simulink model "BLDC_Mathematical_Model"  (R2015a)
settings: Solver=ode45  StartTime=0.0  StopTime=1
values from neighbouring files (symbols this model uses):
  B = 2e-3    (= 0.002)    [BLDC_Mathematical_Model_Script.m]
  J = 5.5e-3    (= 0.0055)    [BLDC_Mathematical_Model_Script.m]
  Ke = 1    [BLDC_Mathematical_Model_Script.m]
  Kt = 1    [BLDC_Mathematical_Model_Script.m]
  L = 9.4e-3    (= 0.0094)    [BLDC_Mathematical_Model_Script.m]
  P = 4    [BLDC_Mathematical_Model_Script.m]
  phi_m = 0.2158    [BLDC_Mathematical_Model_Script.m]
  R = 1.43    [BLDC_Mathematical_Model_Script.m]
  trap = 0.2    [BLDC_Mathematical_Model_Script.m]
settings Model: Creator=Koustubh  LastModifiedBy=Koustubh

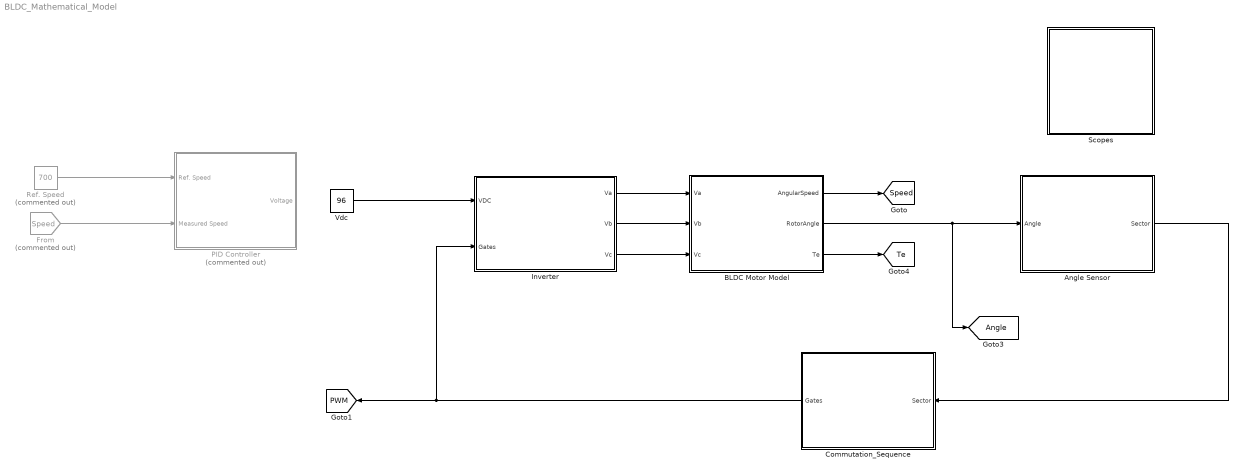
== system BLDC_Mathematical_Model ==
  Angle Sensor : Subsystem
  BLDC Motor Model : Subsystem
      mask Display: image(imread('F:\VAC_2003_MATLAB_Simulink\Practice\BLDC_Mathematical_Model\BLDC_Motor.jpg'))
  Commutation_Sequence : Subsystem
  From : From  Commented=on  GotoTag=Speed  TagVisibility=global
  Inverter : Subsystem
  "PID Controller " : Subsystem  Commented=on
  Ref. Speed : Constant  Commented=on  Value=700
  Scopes : Subsystem
  Vdc : Constant  Value=96
  tag scope: Angle=global, PWM=global, Speed=global, Te=global
  wires:
  BLDC Motor Model/1(AngularSpeed) -> [Speed]
  BLDC Motor Model/2(RotorAngle) -> [Angle], Angle Sensor/1(Angle)
  Angle Sensor/1(Sector) -> Commutation_Sequence/1(Sector)
  Inverter/1(Va) -> BLDC Motor Model/1(Va)
  Inverter/2(Vb) -> BLDC Motor Model/2(Vb)
  Inverter/3(Vc) -> BLDC Motor Model/3(Vc)
  Commutation_Sequence/1(Gates) -> Inverter/2(Gates), [PWM]
  BLDC Motor Model/3(Te) -> [Te]
  From/1 -> "PID Controller "/2(Measured Speed)
  Ref. Speed/1 -> "PID Controller "/1(Ref. Speed)
  Vdc/1 -> Inverter/1(VDC)

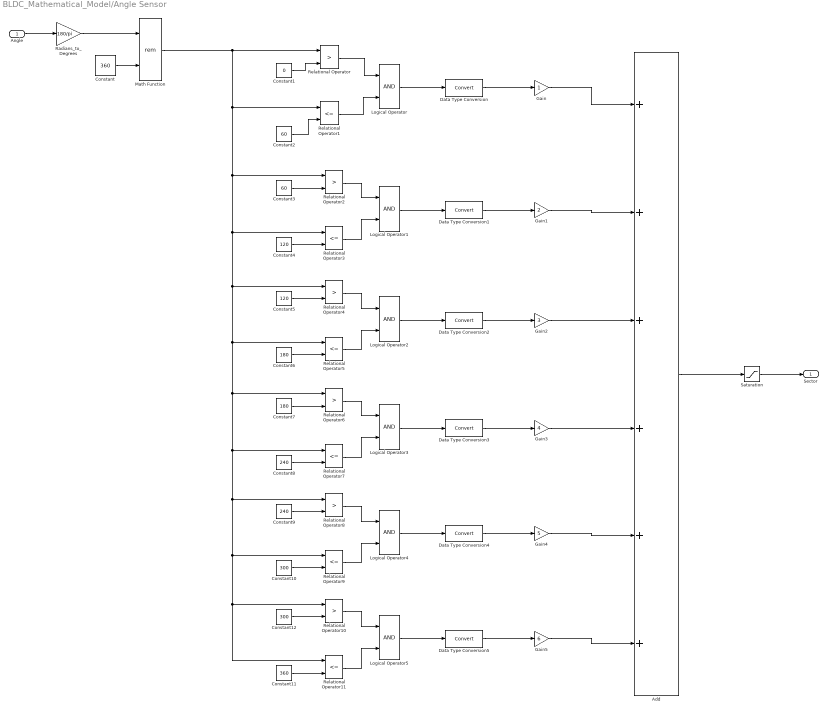
== system BLDC_Mathematical_Model/Angle Sensor ==
  Angle : Inport
  Add : Sum  Inputs=6
  Constant : Constant  Value=360
  Constant1 : Constant  Value=0
  Constant10 : Constant  Value=300
  Constant11 : Constant  Value=360
  Constant12 : Constant  Value=300
  Constant2 : Constant  Value=60
  Constant3 : Constant  Value=60
  Constant4 : Constant  Value=120
  Constant5 : Constant  Value=120
  Constant6 : Constant  Value=180
  Constant7 : Constant  Value=180
  Constant8 : Constant  Value=240
  Constant9 : Constant  Value=240
  Data Type Conversion{,1..5} (6 alike) : DataTypeConversion
  Gain : Gain
  Gain1 : Gain  Gain=2
  Gain2 : Gain  Gain=3
  Gain3 : Gain  Gain=4
  Gain4 : Gain  Gain=5
  Gain5 : Gain  Gain=6
  Logical Operator{,1..5} (6 alike) : Logic  AllPortsSameDT=off  OutDataTypeStr=boolean
  Math Function : Math  Operator=rem  SaturateOnIntegerOverflow=on
  Radians_to_Degrees : Gain  Gain=180/pi
  Relational Operator{,2,4,6,8,10} (6 alike) : RelationalOperator  Operator=>  OutDataTypeStr=boolean
  Relational Operator{1,3,5,7,9,11} (6 alike) : RelationalOperator  Operator=<=  OutDataTypeStr=boolean
  Saturation : Saturate  UpperLimit=6  LowerLimit=1
  Sector : Outport
  wires:
  Constant/1 -> Math Function/2
  Constant1/1 -> Relational Operator/2
  Constant2/1 -> Relational Operator1/2
  Relational Operator/1 -> Logical Operator/1
  Relational Operator1/1 -> Logical Operator/2
  Constant3/1 -> Relational Operator2/2
  Constant4/1 -> Relational Operator3/2
  Relational Operator2/1 -> Logical Operator1/1
  Relational Operator3/1 -> Logical Operator1/2
  Logical Operator/1 -> Data Type Conversion/1
  Data Type Conversion/1 -> Gain/1
  Logical Operator1/1 -> Data Type Conversion1/1
  Data Type Conversion1/1 -> Gain1/1
  Constant5/1 -> Relational Operator4/2
  Constant6/1 -> Relational Operator5/2
  Relational Operator4/1 -> Logical Operator2/1
  Relational Operator5/1 -> Logical Operator2/2
  Logical Operator2/1 -> Data Type Conversion2/1
  Data Type Conversion2/1 -> Gain2/1
  Constant7/1 -> Relational Operator6/2
  Constant8/1 -> Relational Operator7/2
  Relational Operator6/1 -> Logical Operator3/1
  Relational Operator7/1 -> Logical Operator3/2
  Logical Operator3/1 -> Data Type Conversion3/1
  Data Type Conversion3/1 -> Gain3/1
  Constant9/1 -> Relational Operator8/2
  Constant10/1 -> Relational Operator9/2
  Relational Operator8/1 -> Logical Operator4/1
  Relational Operator9/1 -> Logical Operator4/2
  Logical Operator4/1 -> Data Type Conversion4/1
  Data Type Conversion4/1 -> Gain4/1
  Math Function/1 -> Relational Operator4/1, Relational Operator10/1, Relational Operator11/1, Relational Operator9/1, Relational Operator8/1, Relational Operator7/1, Relational Operator6/1, Relational Operator5/1, Relational Operator3/1, Relational Operator2/1, Relational Operator1/1, Relational Operator/1
  Constant12/1 -> Relational Operator10/2
  Constant11/1 -> Relational Operator11/2
  Relational Operator10/1 -> Logical Operator5/1
  Relational Operator11/1 -> Logical Operator5/2
  Logical Operator5/1 -> Data Type Conversion5/1
  Data Type Conversion5/1 -> Gain5/1
  Gain5/1 -> Add/6
  Gain4/1 -> Add/5
  Gain3/1 -> Add/4
  Gain2/1 -> Add/3
  Gain1/1 -> Add/2
  Gain/1 -> Add/1
  Add/1 -> Saturation/1
  Radians_to_Degrees/1 -> Math Function/1
  Angle/1 -> Radians_to_Degrees/1
  Saturation/1 -> Sector/1

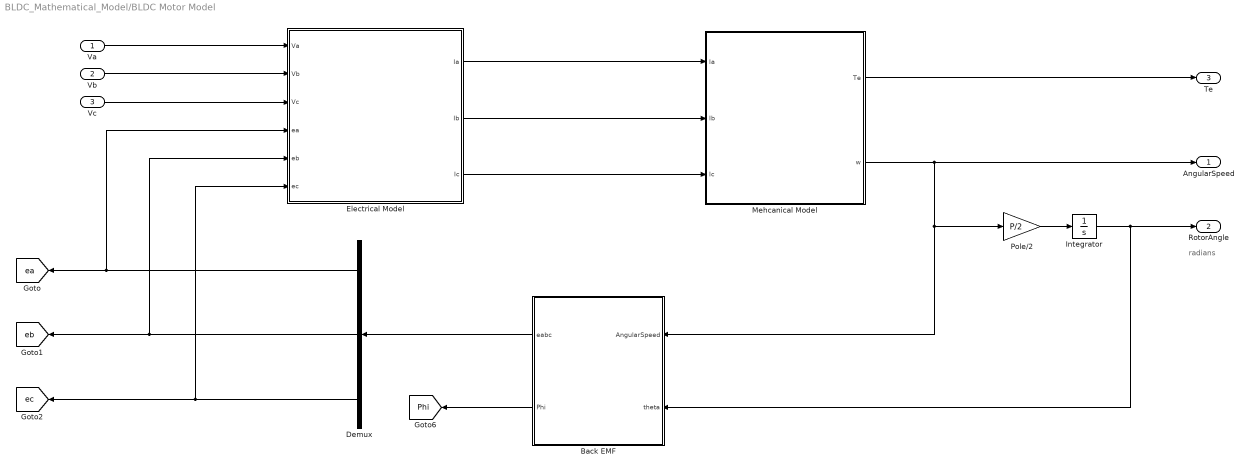
== system BLDC_Mathematical_Model/BLDC Motor Model ==
  note: radians
  Va : Inport
  Vb : Inport  Port=2
  Vc : Inport  Port=3
  Back EMF : Subsystem
  Demux : Demux  Outputs=3
  Electrical Model : Subsystem
  Integrator : Integrator  InitialCondition=0.0000001  UpperSaturationLimit=60  LowerSaturationLimit=-60
  Mehcanical Model : Subsystem
  Pole/2 : Gain  Gain=P/2
  AngularSpeed : Outport
  RotorAngle : Outport  Port=2
  Te : Outport  Port=3
  tag scope: Phi=global, ea=global, eb=global, ec=global
  wires:
  Va/1 -> Electrical Model/1(Va)
  Vb/1 -> Electrical Model/2(Vb)
  Vc/1 -> Electrical Model/3(Vc)
  Electrical Model/3(Ic) -> Mehcanical Model/3(Ic)
  Electrical Model/2(Ib) -> Mehcanical Model/2(Ib)
  Electrical Model/1(Ia) -> Mehcanical Model/1(Ia)
  Integrator/1 -> Back EMF/2(theta), RotorAngle/1
  Back EMF/2(Phi) -> [Phi]
  Pole/2/1 -> Integrator/1
  Back EMF/1(eabc) -> Demux/1
  Demux/1 -> Electrical Model/4(ea), [ea]
  Demux/2 -> Electrical Model/5(eb), [eb]
  Demux/3 -> Electrical Model/6(ec), [ec]
  Mehcanical Model/2(w) -> AngularSpeed/1, Back EMF/1(AngularSpeed), Pole/2/1
  Mehcanical Model/1(Te) -> Te/1

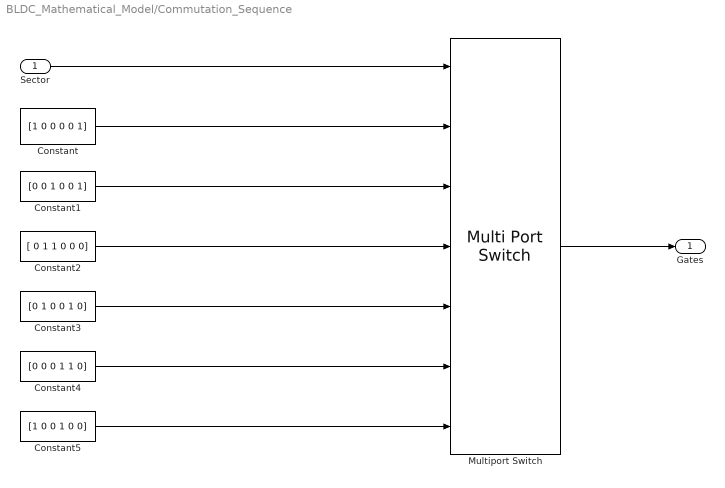
== system BLDC_Mathematical_Model/Commutation_Sequence ==
  Sector : Inport
  Constant : Constant  Value=[1 0 0 0 0 1]
  Constant1 : Constant  Value=[0 0 1 0 0 1]
  Constant2 : Constant  Value=[ 0 1 1 0 0 0]
  Constant3 : Constant  Value=[0 1 0 0 1 0]
  Constant4 : Constant  Value=[0 0 0 1 1 0]
  Constant5 : Constant  Value=[1 0 0 1 0 0]
  Multiport Switch : MultiPortSwitch  Inputs=6  DiagnosticForDefault=None
  Gates : Outport
  wires:
  Sector/1 -> Multiport Switch/1
  Constant/1 -> Multiport Switch/2
  Constant5/1 -> Multiport Switch/7
  Constant4/1 -> Multiport Switch/6
  Constant3/1 -> Multiport Switch/5
  Constant2/1 -> Multiport Switch/4
  Constant1/1 -> Multiport Switch/3
  Multiport Switch/1 -> Gates/1

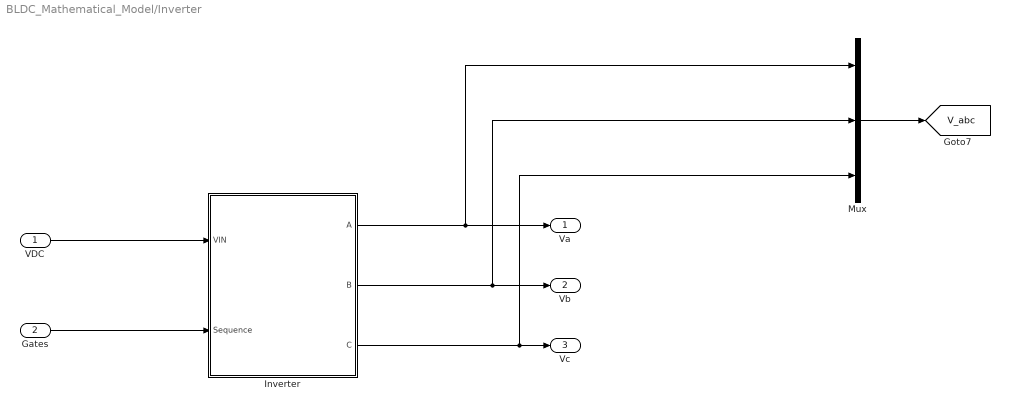
== system BLDC_Mathematical_Model/Inverter ==
  VDC : Inport
  Gates : Inport  Port=2
  Inverter : Subsystem
  Mux : Mux  Inputs=3
  Va : Outport
  Vb : Outport  Port=2
  Vc : Outport  Port=3
  tag scope: V_abc=global
  wires:
  Inverter/3(C) -> Mux/3, Vc/1
  Inverter/2(B) -> Vb/1, Mux/2
  Inverter/1(A) -> Mux/1, Va/1
  Gates/1 -> Inverter/2(Sequence)
  Mux/1 -> [V_abc]
  VDC/1 -> Inverter/1(VIN)

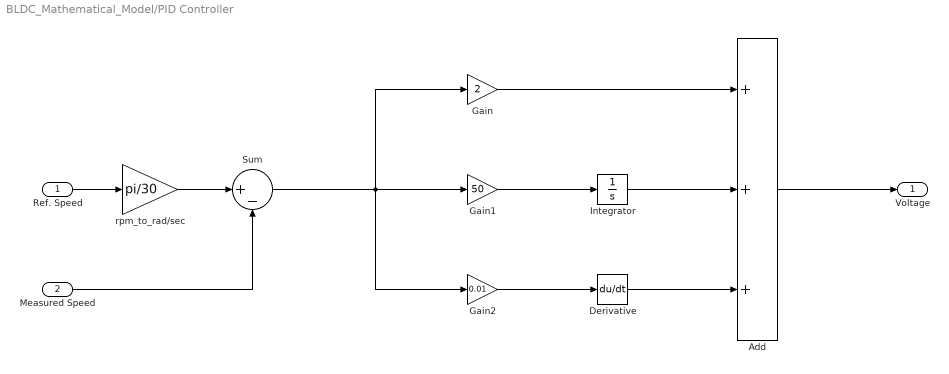
== system BLDC_Mathematical_Model/PID Controller  ==
  Ref. Speed : Inport
  Measured Speed : Inport  Port=2
  Add : Sum  Inputs=+++
  Derivative : Derivative
  Gain : Gain  Gain=2
  Gain1 : Gain  Gain=50
  Gain2 : Gain  Gain=0.01
  Integrator : Integrator
  Sum : Sum  Inputs=|+-
  rpm_to_rad/sec : Gain  Gain=pi/30
  Voltage : Outport
  wires:
  Sum/1 -> Gain/1, Gain2/1, Gain1/1
  Measured Speed/1 -> Sum/2
  Ref. Speed/1 -> rpm_to_rad/sec/1
  rpm_to_rad/sec/1 -> Sum/1
  Gain1/1 -> Integrator/1
  Gain2/1 -> Derivative/1
  Gain/1 -> Add/1
  Integrator/1 -> Add/2
  Derivative/1 -> Add/3
  Add/1 -> Voltage/1

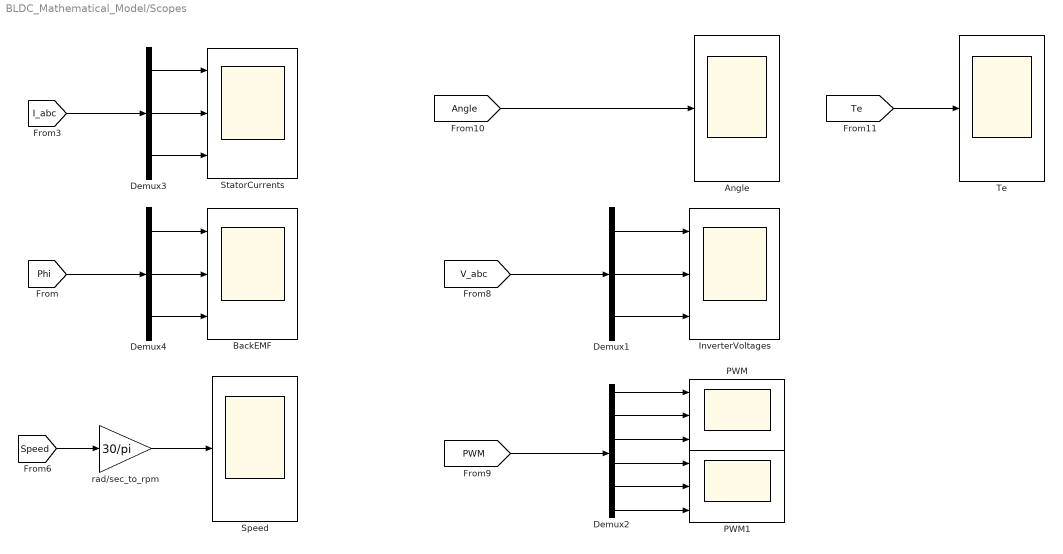
== system BLDC_Mathematical_Model/Scopes ==
  Angle : Scope
      settings: SaveName=ScopeData6
  BackEMF : Scope  NumInputPorts=3
      settings: YMin=-5~-5~-5  YMax=5~5~5  SaveName=ScopeData2
  Demux1 : Demux  Outputs=3
  Demux2 : Demux  Outputs=6
  Demux3 : Demux  Outputs=3
  Demux4 : Demux  Outputs=3
  InverterVoltages : Scope  NumInputPorts=3
      settings: YMin=-5~-5~-5  YMax=5~5~5  SaveName=ScopeData3
  PWM : Scope  NumInputPorts=3
      settings: YMin=-5~-5~-5  YMax=5~5~5  SaveName=ScopeData5
  PWM1 : Scope  NumInputPorts=3
      settings: YMin=-5~-5~-5  YMax=5~5~5  SaveName=ScopeData7
  Speed : Scope
  StatorCurrents : Scope  NumInputPorts=3
      settings: YMin=-5~-5~-5  YMax=5~5~5  SaveName=ScopeData4
  Te : Scope
      settings: SaveName=ScopeData8
  rad/sec_to_rpm : Gain  Gain=30/pi
  wires:
  Demux1/2 -> InverterVoltages/2
  Demux1/1 -> InverterVoltages/1
  Demux1/3 -> InverterVoltages/3
  [V_abc] -> Demux1/1
  [PWM] -> Demux2/1
  Demux2/1 -> PWM/1
  Demux2/2 -> PWM/2
  Demux2/3 -> PWM/3
  Demux2/4 -> PWM1/1
  Demux2/5 -> PWM1/2
  Demux2/6 -> PWM1/3
  [Angle] -> Angle/1
  [Speed] -> rad/sec_to_rpm/1
  rad/sec_to_rpm/1 -> Speed/1
  [Te] -> Te/1
  Demux3/1 -> StatorCurrents/1
  Demux3/2 -> StatorCurrents/2
  Demux3/3 -> StatorCurrents/3
  [I_abc] -> Demux3/1
  Demux4/1 -> BackEMF/1
  Demux4/2 -> BackEMF/2
  Demux4/3 -> BackEMF/3
  [Phi] -> Demux4/1

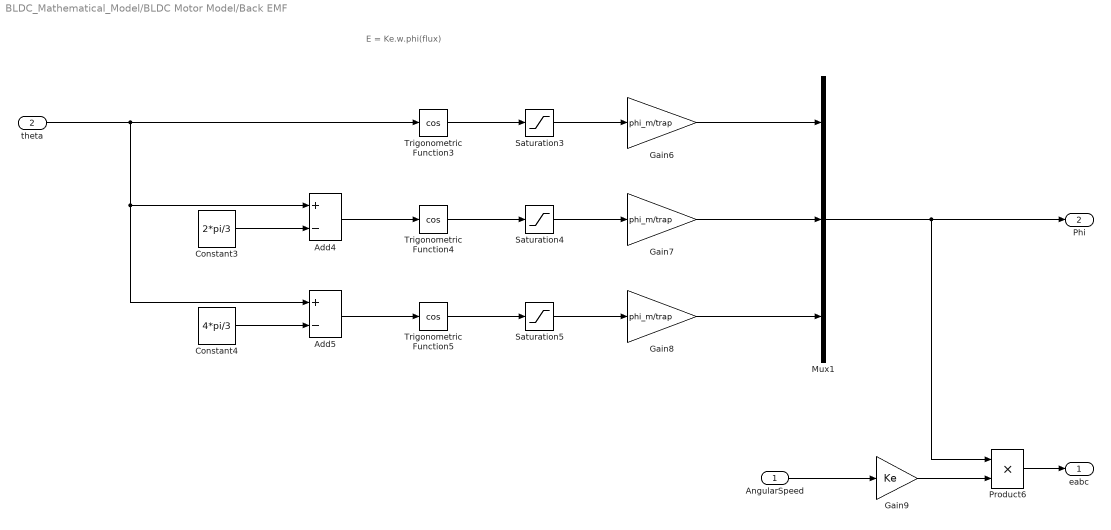
== system BLDC_Mathematical_Model/BLDC Motor Model/Back EMF ==
  note: E = Ke.w.phi(flux)
  AngularSpeed : Inport
  theta : Inport  Port=2
  Add4 : Sum  Inputs=+-
  Add5 : Sum  Inputs=+-
  Constant3 : Constant  Value=2*pi/3
  Constant4 : Constant  Value=4*pi/3
  Gain6 : Gain  Gain=phi_m/trap
  Gain7 : Gain  Gain=phi_m/trap
  Gain8 : Gain  Gain=phi_m/trap
  Gain9 : Gain  Gain=Ke
  Mux1 : Mux  Inputs=3
  Product6 : Product
  Saturation3 : Saturate  UpperLimit=trap  LowerLimit=-trap
  Saturation4 : Saturate  UpperLimit=trap  LowerLimit=-trap
  Saturation5 : Saturate  UpperLimit=trap  LowerLimit=-trap
  Trigonometric Function3 : Trigonometry  Operator=cos
  Trigonometric Function4 : Trigonometry  Operator=cos
  Trigonometric Function5 : Trigonometry  Operator=cos
  eabc : Outport
  Phi : Outport  Port=2
  wires:
  theta/1 -> Trigonometric Function3/1, Add4/1, Add5/1
  Trigonometric Function3/1 -> Saturation3/1
  Trigonometric Function4/1 -> Saturation4/1
  Trigonometric Function5/1 -> Saturation5/1
  Add4/1 -> Trigonometric Function4/1
  Add5/1 -> Trigonometric Function5/1
  Constant3/1 -> Add4/2
  Constant4/1 -> Add5/2
  Saturation3/1 -> Gain6/1
  Saturation4/1 -> Gain7/1
  Saturation5/1 -> Gain8/1
  Gain7/1 -> Mux1/2
  Gain6/1 -> Mux1/1
  Gain8/1 -> Mux1/3
  AngularSpeed/1 -> Gain9/1
  Product6/1 -> eabc/1
  Gain9/1 -> Product6/2
  Mux1/1 -> Product6/1, Phi/1

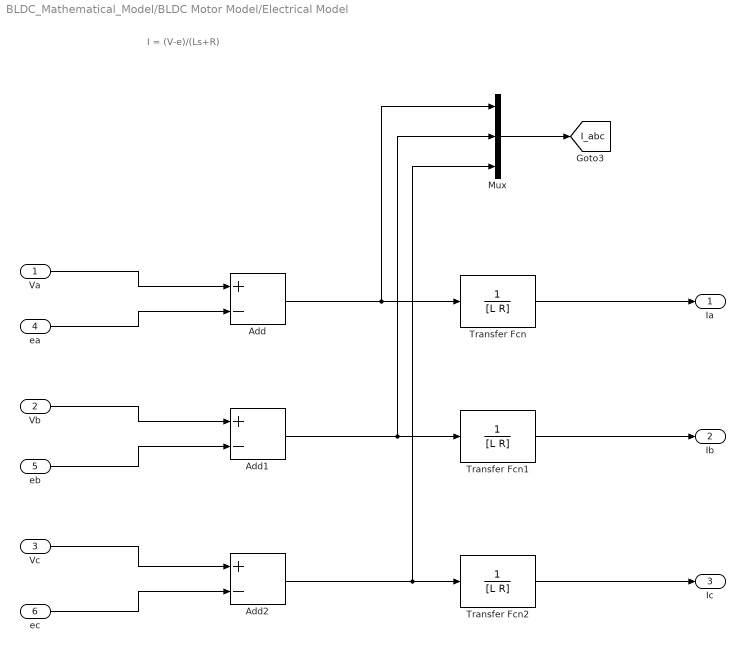
== system BLDC_Mathematical_Model/BLDC Motor Model/Electrical Model ==
  note: I = (V-e)/(Ls+R)
  Va : Inport
  Vb : Inport  Port=2
  Vc : Inport  Port=3
  ea : Inport  Port=4
  eb : Inport  Port=5
  ec : Inport  Port=6
  Add : Sum  Inputs=+-
  Add1 : Sum  Inputs=+-
  Add2 : Sum  Inputs=+-
  Mux : Mux  Inputs=3
  Transfer Fcn : TransferFcn  Denominator=[L R]
  Transfer Fcn1 : TransferFcn  Denominator=[L R]
  Transfer Fcn2 : TransferFcn  Denominator=[L R]
  Ia : Outport
  Ib : Outport  Port=2
  Ic : Outport  Port=3
  tag scope: I_abc=global
  wires:
  Va/1 -> Add/1
  ea/1 -> Add/2
  Vb/1 -> Add1/1
  eb/1 -> Add1/2
  Vc/1 -> Add2/1
  ec/1 -> Add2/2
  Add/1 -> Mux/1, Transfer Fcn/1
  Add1/1 -> Mux/2, Transfer Fcn1/1
  Add2/1 -> Mux/3, Transfer Fcn2/1
  Transfer Fcn/1 -> Ia/1
  Transfer Fcn1/1 -> Ib/1
  Transfer Fcn2/1 -> Ic/1
  Mux/1 -> [I_abc]

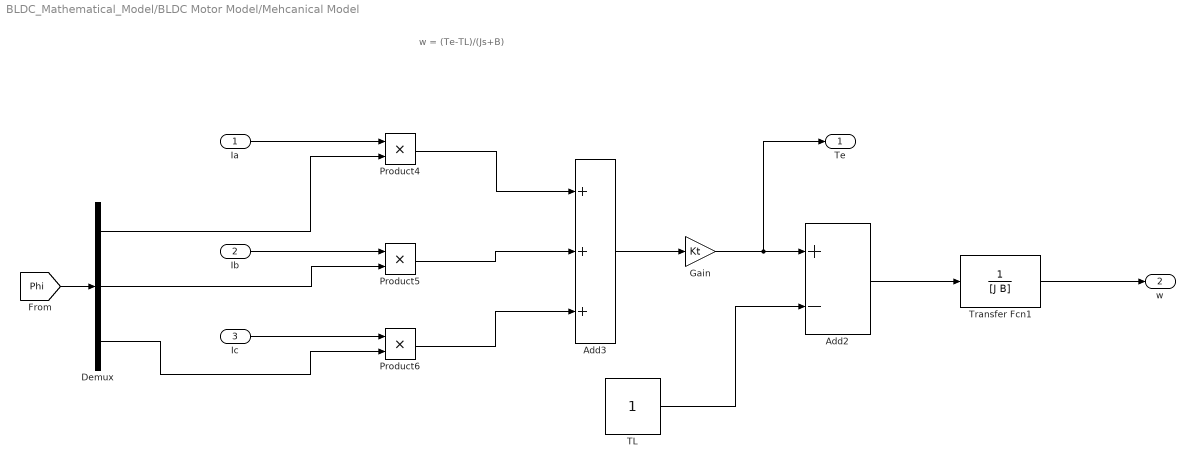
== system BLDC_Mathematical_Model/BLDC Motor Model/Mehcanical Model ==
  note: w = (Te-TL)/(Js+B)
  Ia : Inport
  Ib : Inport  Port=2
  Ic : Inport  Port=3
  Add2 : Sum  Inputs=+-
  Add3 : Sum  Inputs=+++
  Demux : Demux  Outputs=3
  Gain : Gain  Gain=Kt
  Product4 : Product
  Product5 : Product
  Product6 : Product
  TL : Constant
  Transfer Fcn1 : TransferFcn  Denominator=[J B]
  Te : Outport
  w : Outport  Port=2
  wires:
  Add2/1 -> Transfer Fcn1/1
  Transfer Fcn1/1 -> w/1
  Add3/1 -> Gain/1
  TL/1 -> Add2/2
  Gain/1 -> Te/1, Add2/1
  [Phi] -> Demux/1
  Ib/1 -> Product5/1
  Ia/1 -> Product4/1
  Ic/1 -> Product6/1
  Demux/1 -> Product4/2
  Demux/2 -> Product5/2
  Demux/3 -> Product6/2
  Product4/1 -> Add3/1
  Product5/1 -> Add3/2
  Product6/1 -> Add3/3

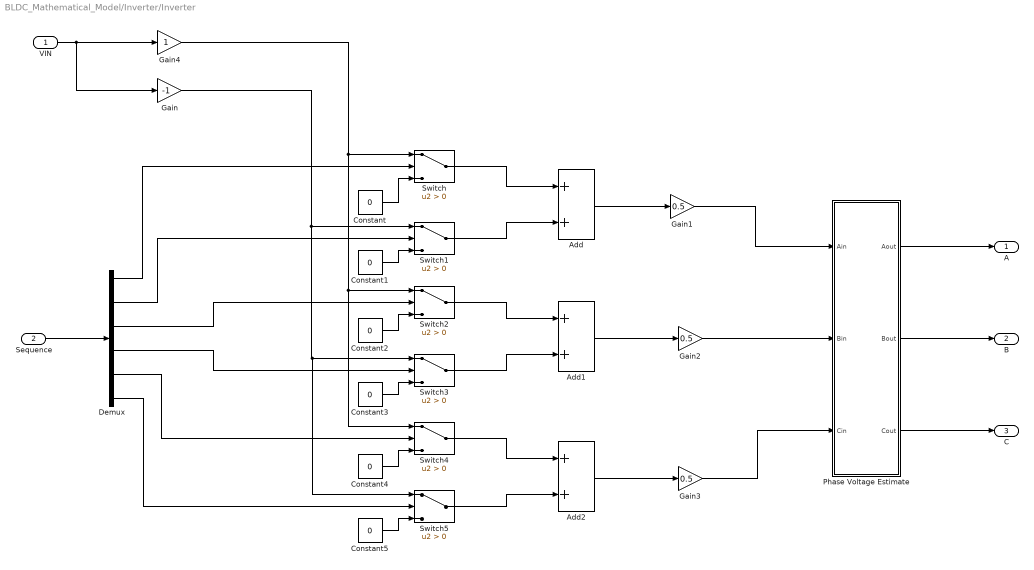
== system BLDC_Mathematical_Model/Inverter/Inverter ==
  VIN : Inport
  Sequence : Inport  Port=2
  Add : Sum
  Add1 : Sum
  Add2 : Sum
  Constant{,1..5} (6 alike) : Constant  Value=0
  Demux : Demux  Outputs=6
  Gain : Gain  Gain=-1
  Gain1 : Gain  Gain=0.5
  Gain2 : Gain  Gain=0.5
  Gain3 : Gain  Gain=0.5
  Gain4 : Gain
  Phase Voltage Estimate : Subsystem
  Switch{,1..5} (6 alike) : Switch  Criteria=u2 > Threshold
  A : Outport
  B : Outport  Port=2
  C : Outport  Port=3
  wires:
  VIN/1 -> Gain/1, Gain4/1
  Gain/1 -> Switch1/1, Switch5/1, Switch3/1
  Sequence/1 -> Demux/1
  Demux/1 -> Switch/2
  Demux/2 -> Switch1/2
  Demux/3 -> Switch2/2
  Demux/4 -> Switch3/2
  Demux/5 -> Switch4/2
  Demux/6 -> Switch5/2
  Constant/1 -> Switch/3
  Constant1/1 -> Switch1/3
  Constant2/1 -> Switch2/3
  Constant3/1 -> Switch3/3
  Constant4/1 -> Switch4/3
  Constant5/1 -> Switch5/3
  Switch/1 -> Add/1
  Switch1/1 -> Add/2
  Switch2/1 -> Add1/1
  Switch3/1 -> Add1/2
  Switch4/1 -> Add2/1
  Switch5/1 -> Add2/2
  Add/1 -> Gain1/1
  Add1/1 -> Gain2/1
  Add2/1 -> Gain3/1
  Gain2/1 -> Phase Voltage Estimate/2(Bin)
  Gain1/1 -> Phase Voltage Estimate/1(Ain)
  Gain3/1 -> Phase Voltage Estimate/3(Cin)
  Phase Voltage Estimate/1(Aout) -> A/1
  Phase Voltage Estimate/2(Bout) -> B/1
  Phase Voltage Estimate/3(Cout) -> C/1
  Gain4/1 -> Switch4/1, Switch2/1, Switch/1

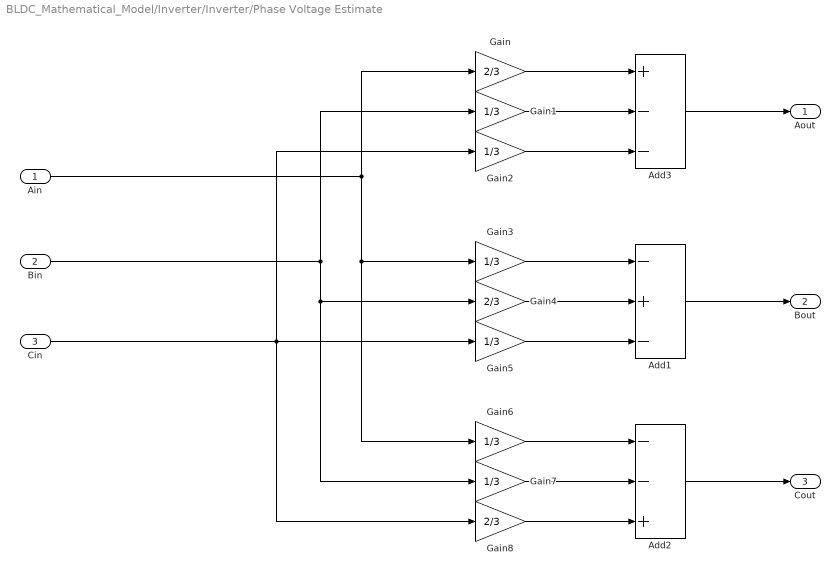
== system BLDC_Mathematical_Model/Inverter/Inverter/Phase Voltage Estimate ==
  Ain : Inport
  Bin : Inport  Port=2
  Cin : Inport  Port=3
  Add1 : Sum  Inputs=-+-
  Add2 : Sum  Inputs=--+
  Add3 : Sum  Inputs=+--
  Gain : Gain  Gain=2/3
  Gain{1..3,5..7} (6 alike) : Gain  Gain=1/3
  Gain4 : Gain  Gain=2/3
  Gain8 : Gain  Gain=2/3
  Aout : Outport
  Bout : Outport  Port=2
  Cout : Outport  Port=3
  wires:
  Gain/1 -> Add3/1
  Gain1/1 -> Add3/2
  Gain2/1 -> Add3/3
  Gain3/1 -> Add1/1
  Gain4/1 -> Add1/2
  Gain5/1 -> Add1/3
  Gain6/1 -> Add2/1
  Gain7/1 -> Add2/2
  Gain8/1 -> Add2/3
  Ain/1 -> Gain/1, Gain6/1, Gain3/1
  Bin/1 -> Gain7/1, Gain4/1, Gain1/1
  Cin/1 -> Gain8/1, Gain5/1, Gain2/1
  Add2/1 -> Cout/1
  Add1/1 -> Bout/1
  Add3/1 -> Aout/1
